simulink library "fzgbib"  (Simulink 4.1.1)
values from neighbouring files (symbols this model uses):
  a_Fzg_max = 2    [PedalInterp_para.m]
  a_Fzg_min = -2    [PedalInterp_para.m]
  gang0 = 1    [PedalInterp_para.m]
  gang_vec = [1 2 3 4]    [PedalInterp_para.m]
  lambda_gang = [1.3 1.25  1.17  1.05]    [PedalInterp_para.m]
  M_Br_max = 4000    [PedalInterp_para.m]
undefined symbols (not defined in the file or in its folder): A, cw, gang, i_d, i_g, m_ab_100pro, m_ab_70pro, m_Fzg, M_mot_max, M_mot_min, n_mot0, n_mot_max, n_mot_min, p_anteil, r_dyn, rho, t_sch, v_bereich, v_Fzg_ms0
libraries: simulink3 x1
(part 1 of 2)
settings Model: LastModifiedBy=MCONRAD

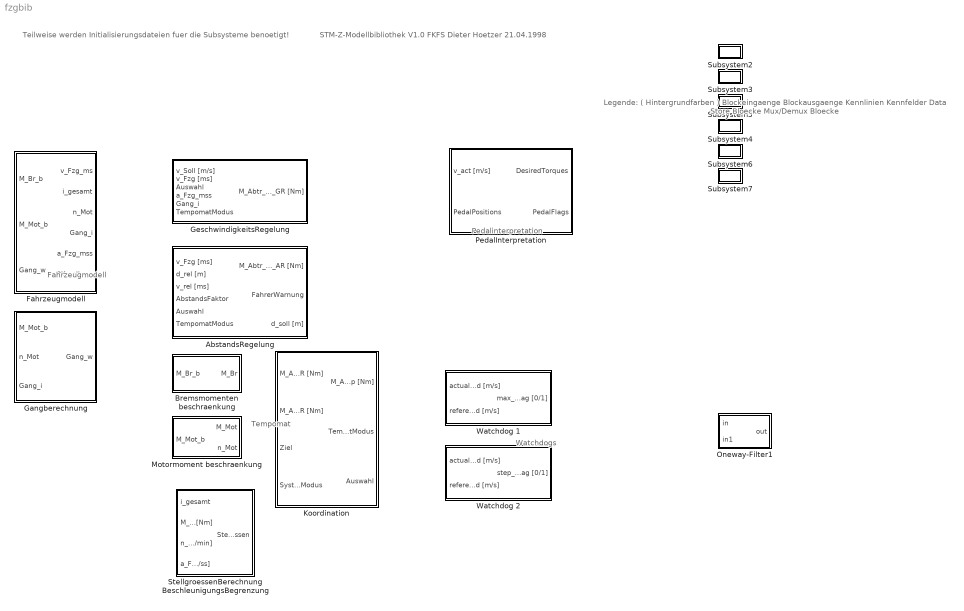
== system fzgbib ==
  note: STM-Z-Modellbibliothek V1.0
      | FKFS
      | Dieter Hoetzer
      | 21.04.1998
  note: Legende:         ( Hintergrundfarben )
      |
      |
      |                      Blockeingaenge
      |
      |                     Blockausgaenge
      |
      |                    Kennlinien
      |
      |                     Kennfelder
      |
      |                     Data Store Bloecke
      |
      |                     Mux/Demux Bloecke
  note: Fahrzeugmodell
  note: Tempomat
  note: Pedalinterpretation
  note: Watchdogs
  note: Teilweise werden Initialisierungsdateien fuer
      | die Subsysteme benoetigt!
  AbstandsRegelung : Subsystem
      settings: RTWFcnNameOpts=Auto  RTWFileNameOpts=Auto
  Bremsmomenten beschraenkung : Subsystem  Orientation=left
      settings: RTWFcnNameOpts=Auto  RTWFileNameOpts=Auto
  Fahrzeugmodell : Subsystem
      settings: RTWFcnNameOpts=Auto  RTWFileNameOpts=Auto
  Gangberechnung : Subsystem
      settings: RTWFcnNameOpts=Auto  RTWFileNameOpts=Auto
  GeschwindigkeitsRegelung : Subsystem
      settings: RTWFcnNameOpts=Auto  RTWFileNameOpts=Auto
  Koordination : Subsystem
      settings: RTWFcnNameOpts=Auto  RTWFileNameOpts=Auto
  Motormoment beschraenkung : Subsystem  Orientation=left
      settings: RTWFcnNameOpts=Auto  RTWFileNameOpts=Auto
  Oneway-Filter1 : Subsystem  mask(Oneway Filter){zk=2}
      mask prompts: zk "Filterkonstante"
      mask help: Filtert Signal mit Zeitkonstante zk nur, wenn kein Sprung auf Null von oben.
      settings: RTWFcnNameOpts=Auto  RTWFileNameOpts=Auto
      mask Display: plot(0,0,100,100,[0 10 20 30 40 50 60 60 100],[0 0 30 50 60 65 67 0 0])
  PedalInterpretation : Subsystem
      settings: RTWFcnNameOpts=Auto  RTWFileNameOpts=Auto
  StellgroessenBerechnung BeschleunigungsBegrenzung : Subsystem
      settings: RTWFcnNameOpts=Auto  RTWFileNameOpts=Auto
  Subsystem2 : Subsystem
      settings: RTWFcnNameOpts=Auto  RTWFileNameOpts=Auto
  Subsystem3 : Subsystem
      settings: RTWFcnNameOpts=Auto  RTWFileNameOpts=Auto
  Subsystem4 : Subsystem
      settings: RTWFcnNameOpts=Auto  RTWFileNameOpts=Auto
  Subsystem5 : Subsystem
      settings: RTWFcnNameOpts=Auto  RTWFileNameOpts=Auto
  Subsystem6 : Subsystem
      settings: RTWFcnNameOpts=Auto  RTWFileNameOpts=Auto
  Subsystem7 : Subsystem
      settings: RTWFcnNameOpts=Auto  RTWFileNameOpts=Auto
  Watchdog 1 : Subsystem
      settings: RTWFcnNameOpts=Auto  RTWFileNameOpts=Auto
  Watchdog 2 : Subsystem
      settings: RTWFcnNameOpts=Auto  RTWFileNameOpts=Auto

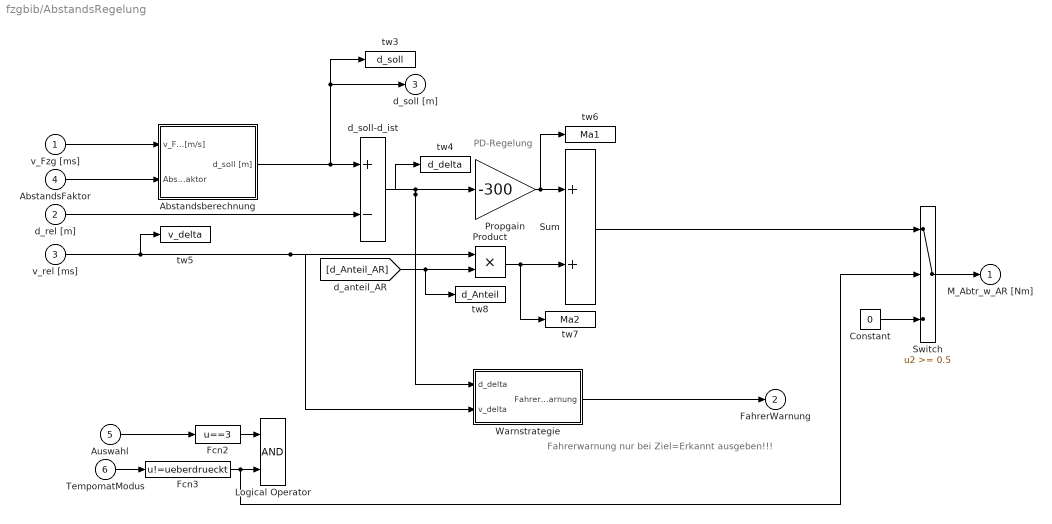
== system fzgbib/AbstandsRegelung ==
  note: PD-Regelung
  note: Fahrerwarnung
      | nur bei Ziel=Erkannt
      | ausgeben!!!
  v_Fzg [ms] : Inport  Port=1  LatchInput=off
  d_rel [m] : Inport  Port=2  LatchInput=off
  v_rel [ms] : Inport  Port=3  LatchInput=off
  AbstandsFaktor : Inport  Port=4  LatchInput=off
  Auswahl : Inport  Port=5  LatchInput=off
  TempomatModus : Inport  Port=6  LatchInput=off
  "Abstandsberechnung " : Subsystem
      settings: RTWFcnNameOpts=Auto  RTWFileNameOpts=Auto
  Constant : Constant  Value=0
  Fcn2 : Fcn  Expr=u==3
  Fcn3 : Fcn  Expr=u!=ueberdrueckt
  Logical Operator : Logic  Operator=AND  Inputs=2
  Product : Product  Inputs=2  Multiplication=Element-wise(.*)  SaturateOnIntegerOverflow=on
  Propgain : Gain  Gain=-300  Multiplication=Element-wise(K.*u)  SaturateOnIntegerOverflow=on
  Sum : Sum  Inputs=++  SaturateOnIntegerOverflow=on
  Switch : Switch  Threshold=0.5
  Warnstrategie : Subsystem
      settings: RTWFcnNameOpts=Auto  RTWFileNameOpts=Auto
  d_soll-d_ist : Sum  Inputs=+-  SaturateOnIntegerOverflow=on
  tw3 : ToWorkspace  VariableName=d_soll  SampleTime=0  SaveFormat=Array
      settings: MaxDataPoints=speicher
  tw4 : ToWorkspace  VariableName=d_delta  SampleTime=0  SaveFormat=Array
      settings: MaxDataPoints=speicher
  tw5 : ToWorkspace  VariableName=v_delta  SampleTime=0  SaveFormat=Array
      settings: MaxDataPoints=speicher
  tw6 : ToWorkspace  VariableName=Ma1  SampleTime=0  SaveFormat=Array
      settings: MaxDataPoints=speicher
  tw7 : ToWorkspace  VariableName=Ma2  SampleTime=0  SaveFormat=Array
      settings: MaxDataPoints=speicher
  tw8 : ToWorkspace  VariableName=d_Anteil  SampleTime=0  SaveFormat=Array
      settings: MaxDataPoints=speicher
  M_Abtr_w_AR [Nm] : Outport  Port=1  InitialOutput=0
  FahrerWarnung : Outport  Port=2  InitialOutput=0
  d_soll [m] : Outport  Port=3  InitialOutput=0
  wires:
  Fcn3/1 -> Switch/2, Logical Operator/2
  TempomatModus/1 -> Fcn3/1
  Fcn2/1 -> Logical Operator/1
  Auswahl/1 -> Fcn2/1
  Sum/1 -> Switch/1
  Switch/1 -> M_Abtr_w_AR [Nm]/1
  Constant/1 -> Switch/3
  Product/1 -> Sum/2, tw7/1
  Propgain/1 -> tw6/1, Sum/1
  d_soll-d_ist/1 -> tw4/1, Propgain/1, Warnstrategie/1(d_delta)
  Warnstrategie/1(FahrerWarnung) -> FahrerWarnung/1
  "Abstandsberechnung "/1(d_soll [m]) -> d_soll-d_ist/1, d_soll [m]/1, tw3/1
  d_rel [m]/1 -> d_soll-d_ist/2
  v_Fzg [ms]/1 -> "Abstandsberechnung "/1(v_Fzg [m/s])
  AbstandsFaktor/1 -> "Abstandsberechnung "/2(AbstandsFaktor)
  v_rel [ms]/1 -> tw5/1, Product/1, Warnstrategie/2(v_delta)
  [d_Anteil_AR] -> Product/2, tw8/1

== system fzgbib/Bremsmomenten beschraenkung ==
  M_Br : Inport  Port=1  LatchInput=off
  Maximales  Bremsmoment : Saturate  UpperLimit=M_Br_max  LowerLimit=0  LinearizeAsGain=on
  M_Br_b : Outport  Port=1  InitialOutput=0
  wires:
  M_Br/1 -> Maximales  Bremsmoment/1
  Maximales  Bremsmoment/1 -> M_Br_b/1

== system fzgbib/Fahrzeugmodell ==
  M_Br_b : Inport  Port=1  LatchInput=off
  M_Mot_b : Inport  Port=2  LatchInput=off
  Gang_w : Inport  Port=3  LatchInput=off
  Drosselklappenstellung : Subsystem
      settings: RTWFcnNameOpts=Auto  RTWFileNameOpts=Auto
  Fahrwiderstaende : Subsystem
      settings: RTWFcnNameOpts=Auto  RTWFileNameOpts=Auto
  Fahrzeugdynamik : Subsystem
      settings: RTWFcnNameOpts=Auto  RTWFileNameOpts=Auto
  tw6 : ToWorkspace  VariableName=v_Fzg_kmh  SampleTime=0  SaveFormat=Array
      settings: MaxDataPoints=speicher
  v_Fzg_ms : Outport  Port=1  InitialOutput=0
  i_gesamt : Outport  Port=2  InitialOutput=0
  n_Mot : Outport  Port=3  InitialOutput=0
  Gang_i : Outport  Port=4  InitialOutput=0
  a_Fzg_mss : Outport  Port=5  InitialOutput=0
  "DK_Stellung " : Outport  Port=6  InitialOutput=0
  wires:
  Fahrwiderstaende/5(i_gesamt) -> i_gesamt/1, Fahrzeugdynamik/5(i_gesamt)
  M_Br_b/1 -> Fahrwiderstaende/2(M_Br_b)
  Gang_w/1 -> Fahrwiderstaende/3(Gang_w)
  M_Mot_b/1 -> Fahrwiderstaende/1(M_Mot_b), Drosselklappenstellung/2(M_Mot_b)
  Fahrwiderstaende/3(F_R) -> Fahrzeugdynamik/3(F_R)
  Fahrwiderstaende/2(F_L) -> Fahrzeugdynamik/2(F_L)
  Fahrwiderstaende/4(F_Brems) -> Fahrzeugdynamik/4(F_Brems)
  Fahrwiderstaende/1(F_A) -> Fahrzeugdynamik/1(F_A)
  Drosselklappenstellung/1(DK_Stellung [Grad]) -> "DK_Stellung "/1
  Fahrzeugdynamik/2(v_Fzg_ms) -> v_Fzg_ms/1, Fahrwiderstaende/4(v_Fzg_ms)
  Fahrzeugdynamik/3(n_Mot) -> n_Mot/1, Drosselklappenstellung/1(n_mot)
  Fahrwiderstaende/6(Gang_i) -> Fahrzeugdynamik/6(Gang_i), Gang_i/1
  Fahrzeugdynamik/1(v_Fzg_kmh) -> tw6/1
  Fahrzeugdynamik/4(a_Fzg_mss) -> a_Fzg_mss/1
  Fahrwiderstaende/7(schalt_l) -> Drosselklappenstellung/3(schalt_l)

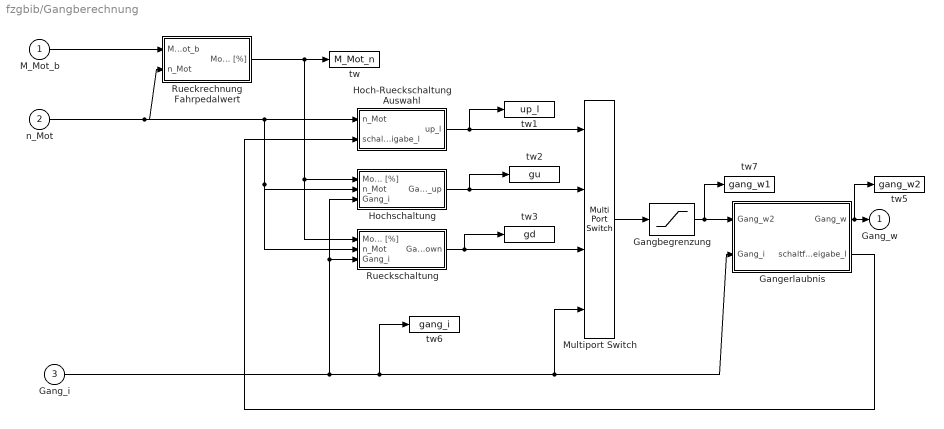
== system fzgbib/Gangberechnung ==
  M_Mot_b : Inport  Port=1  LatchInput=off
  n_Mot : Inport  Port=2  LatchInput=off
  Gang_i : Inport  Port=3  LatchInput=off
  Gangbegrenzung : Saturate  UpperLimit=4  LowerLimit=1  LinearizeAsGain=on
  Gangerlaubnis : Subsystem
      settings: RTWFcnNameOpts=Auto  RTWFileNameOpts=Auto
  Hoch-Rueckschaltung Auswahl : Subsystem
      settings: RTWFcnNameOpts=Auto  RTWFileNameOpts=Auto
  Hochschaltung : Subsystem
      settings: RTWFcnNameOpts=Auto  RTWFileNameOpts=Auto
  Multiport Switch : MultiPortSwitch  Inputs=3
  Rueckrechnung Fahrpedalwert : Subsystem
      settings: RTWFcnNameOpts=Auto  RTWFileNameOpts=Auto
  Rueckschaltung : Subsystem
      settings: RTWFcnNameOpts=Auto  RTWFileNameOpts=Auto
  tw : ToWorkspace  VariableName=M_Mot_n  SampleTime=0  SaveFormat=Array
      settings: MaxDataPoints=speicher
  tw1 : ToWorkspace  VariableName=up_l  SampleTime=0  SaveFormat=Array
      settings: MaxDataPoints=speicher
  tw2 : ToWorkspace  VariableName=gu  SampleTime=0  SaveFormat=Array
      settings: MaxDataPoints=speicher
  tw3 : ToWorkspace  VariableName=gd  SampleTime=0  SaveFormat=Array
      settings: MaxDataPoints=speicher
  tw5 : ToWorkspace  VariableName=gang_w2  SampleTime=0  SaveFormat=Array
      settings: MaxDataPoints=speicher
  tw6 : ToWorkspace  VariableName=gang_i  SampleTime=0  SaveFormat=Array
      settings: MaxDataPoints=speicher
  tw7 : ToWorkspace  VariableName=gang_w1  SampleTime=0  SaveFormat=Array
      settings: MaxDataPoints=speicher
  Gang_w : Outport  Port=1  InitialOutput=0
  wires:
  Gang_i/1 -> tw6/1, Multiport Switch/4, Gangerlaubnis/2(Gang_i), Rueckschaltung/3(Gang_i), Hochschaltung/3(Gang_i)
  Gangerlaubnis/2(schaltfreigabe_l) -> Hoch-Rueckschaltung Auswahl/2(schaltfreigabe_l)
  Gangbegrenzung/1 -> tw7/1, Gangerlaubnis/1(Gang_w2)
  Hoch-Rueckschaltung Auswahl/1(up_l) -> tw1/1, Multiport Switch/1
  Hochschaltung/1(Gang_up) -> tw2/1, Multiport Switch/2
  Gangerlaubnis/1(Gang_w) -> tw5/1, Gang_w/1
  Multiport Switch/1 -> Gangbegrenzung/1
  M_Mot_b/1 -> Rueckrechnung Fahrpedalwert/1(M_Mot_b)
  n_Mot/1 -> Rueckrechnung Fahrpedalwert/2(n_Mot), Hoch-Rueckschaltung Auswahl/1(n_Mot), Hochschaltung/2(n_Mot), Rueckschaltung/2(n_Mot)
  Rueckrechnung Fahrpedalwert/1(Motormoment [%]) -> tw/1, Hochschaltung/1(Motormoment [%]), Rueckschaltung/1(Motormoment [%])
  Rueckschaltung/1(Gang_down) -> Multiport Switch/3, tw3/1

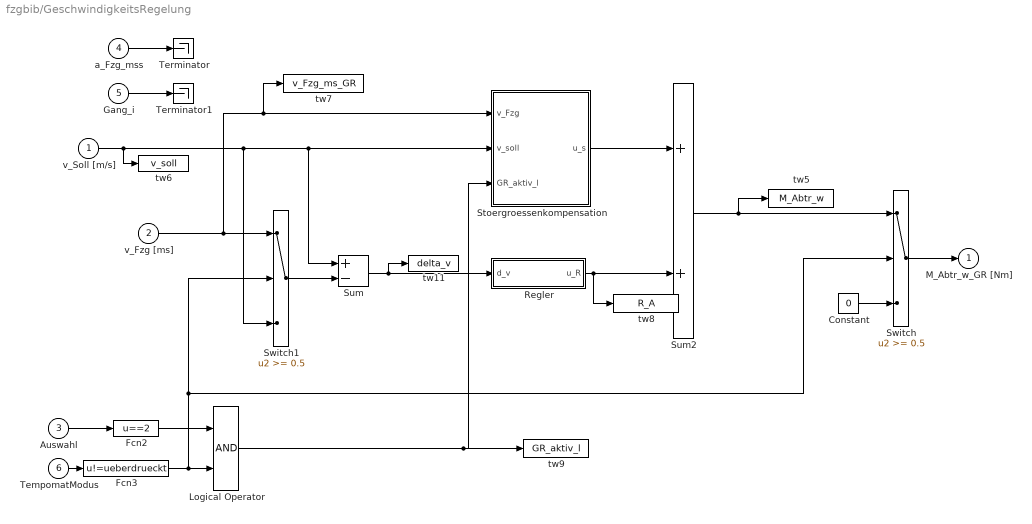
== system fzgbib/GeschwindigkeitsRegelung ==
  v_Soll [m/s] : Inport  Port=1  LatchInput=off
  v_Fzg [ms] : Inport  Port=2  LatchInput=off
  Auswahl : Inport  Port=3  LatchInput=off
  a_Fzg_mss : Inport  Port=4  LatchInput=off
  Gang_i : Inport  Port=5  LatchInput=off
  TempomatModus : Inport  Port=6  LatchInput=off
  Constant : Constant  Value=0
  Fcn2 : Fcn  Expr=u==2
  Fcn3 : Fcn  Expr=u!=ueberdrueckt
  Logical Operator : Logic  Operator=AND  Inputs=2
  Regler : Subsystem
      settings: RTWFcnNameOpts=Auto  RTWFileNameOpts=Auto
  Stoergroessenkompensation : Subsystem
      settings: RTWFcnNameOpts=Auto  RTWFileNameOpts=Auto
  Sum : Sum  Inputs=+-  SaturateOnIntegerOverflow=on
  Sum2 : Sum  Inputs=2  SaturateOnIntegerOverflow=on
  Switch : Switch  Threshold=0.5
  Switch1 : Switch  Threshold=0.5
  Terminator : Terminator
  Terminator1 : Terminator
  tw11 : ToWorkspace  VariableName=delta_v  SampleTime=0  SaveFormat=Array
      settings: MaxDataPoints=speicher
  tw5 : ToWorkspace  VariableName=M_Abtr_w  SampleTime=0  SaveFormat=Array
      settings: MaxDataPoints=speicher
  tw6 : ToWorkspace  VariableName=v_soll  SampleTime=0  SaveFormat=Array
      settings: MaxDataPoints=speicher
  tw7 : ToWorkspace  VariableName=v_Fzg_ms_GR  SampleTime=0  SaveFormat=Array
      settings: MaxDataPoints=speicher
  tw8 : ToWorkspace  VariableName=R_A  SampleTime=0  SaveFormat=Array
      settings: MaxDataPoints=speicher
  tw9 : ToWorkspace  VariableName=GR_aktiv_l  SampleTime=0  SaveFormat=Array
      settings: MaxDataPoints=speicher
  M_Abtr_w_GR [Nm] : Outport  Port=1  InitialOutput=0
  wires:
  v_Soll [m/s]/1 -> Stoergroessenkompensation/2(v_soll), Sum/1, Switch1/3, tw6/1
  Sum2/1 -> tw5/1, Switch/1
  Switch/1 -> M_Abtr_w_GR [Nm]/1
  Fcn3/1 -> Switch/2, Switch1/2, Logical Operator/2
  TempomatModus/1 -> Fcn3/1
  Auswahl/1 -> Fcn2/1
  Fcn2/1 -> Logical Operator/1
  Switch1/1 -> Sum/2
  Constant/1 -> Switch/3
  Sum/1 -> Regler/1(d_v), tw11/1
  v_Fzg [ms]/1 -> Switch1/1, Stoergroessenkompensation/1(v_Fzg), tw7/1
  Stoergroessenkompensation/1(u_s) -> Sum2/1
  a_Fzg_mss/1 -> Terminator/1
  Gang_i/1 -> Terminator1/1
  Regler/1("u_R ") -> Sum2/2, tw8/1
  Logical Operator/1 -> Stoergroessenkompensation/3(GR_aktiv_l), tw9/1

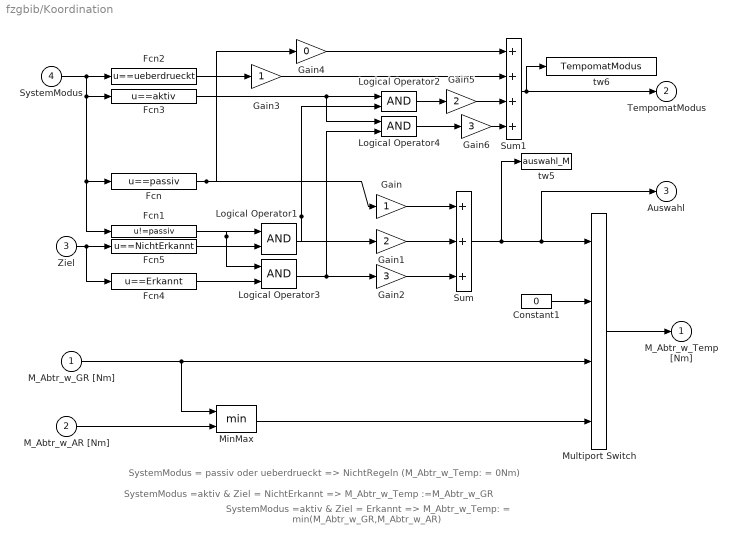
== system fzgbib/Koordination ==
  note: SystemModus = passiv oder ueberdrueckt => NichtRegeln (M_Abtr_w_Temp: = 0Nm)
  note: SystemModus =aktiv & Ziel = Erkannt => M_Abtr_w_Temp: = min(M_Abtr_w_GR,M_Abtr_w_AR)
  note: SystemModus =aktiv & Ziel = NichtErkannt => M_Abtr_w_Temp :=M_Abtr_w_GR
  M_Abtr_w_GR [Nm] : Inport  Port=1  LatchInput=off
  M_Abtr_w_AR [Nm] : Inport  Port=2  LatchInput=off
  Ziel : Inport  Port=3  LatchInput=off
  SystemModus : Inport  Port=4  LatchInput=off
  Constant1 : Constant  Value=0
  Fcn : Fcn  Expr=u==passiv
  Fcn1 : Fcn  Expr=u!=passiv
  Fcn2 : Fcn  Expr=u==ueberdrueckt
  Fcn3 : Fcn  Expr=u==aktiv
  Fcn4 : Fcn  Expr=u==Erkannt
  Fcn5 : Fcn  Expr=u==NichtErkannt
  Gain : Gain  Gain=1  Multiplication=Element-wise(K.*u)  SaturateOnIntegerOverflow=on
  Gain1 : Gain  Gain=2  Multiplication=Element-wise(K.*u)  SaturateOnIntegerOverflow=on
  Gain2 : Gain  Gain=3  Multiplication=Element-wise(K.*u)  SaturateOnIntegerOverflow=on
  Gain3 : Gain  Gain=1  Multiplication=Element-wise(K.*u)  SaturateOnIntegerOverflow=on
  Gain4 : Gain  Gain=0  Multiplication=Element-wise(K.*u)  SaturateOnIntegerOverflow=on
  Gain5 : Gain  Gain=2  Multiplication=Element-wise(K.*u)  SaturateOnIntegerOverflow=on
  Gain6 : Gain  Gain=3  Multiplication=Element-wise(K.*u)  SaturateOnIntegerOverflow=on
  Logical Operator{1..4} (4 alike) : Logic  Operator=AND  Inputs=2
  MinMax : MinMax  Function=min  Inputs=2
  Multiport Switch : MultiPortSwitch  Inputs=3
  Sum : Sum  Inputs=+++  SaturateOnIntegerOverflow=on
  Sum1 : Sum  Inputs=4  SaturateOnIntegerOverflow=on
  tw5 : ToWorkspace  VariableName=auswahl_M  SampleTime=0  SaveFormat=Array
      settings: MaxDataPoints=speicher
  tw6 : ToWorkspace  VariableName=TempomatModus  SampleTime=0  SaveFormat=Array
      settings: MaxDataPoints=speicher
  M_Abtr_w_Temp [Nm] : Outport  Port=1  InitialOutput=0
  TempomatModus : Outport  Port=2  InitialOutput=0
  Auswahl : Outport  Port=3  InitialOutput=0
  wires:
  M_Abtr_w_GR [Nm]/1 -> MinMax/1, Multiport Switch/3
  SystemModus/1 -> Fcn1/1, Fcn/1, Fcn3/1, Fcn2/1
  Ziel/1 -> Fcn4/1, Fcn5/1
  Logical Operator3/1 -> Logical Operator4/2, Gain2/1
  Fcn3/1 -> Logical Operator2/1, Logical Operator4/1
  Sum/1 -> tw5/1, Multiport Switch/1, Auswahl/1
  Multiport Switch/1 -> M_Abtr_w_Temp [Nm]/1
  MinMax/1 -> Multiport Switch/4
  Constant1/1 -> Multiport Switch/2
  Gain4/1 -> Sum1/1
  Fcn/1 -> Gain4/1, Gain/1
  Gain3/1 -> Sum1/2
  Fcn2/1 -> Gain3/1
  M_Abtr_w_AR [Nm]/1 -> MinMax/2
  Fcn4/1 -> Logical Operator3/2
  Fcn1/1 -> Logical Operator1/1, Logical Operator3/1
  Fcn5/1 -> Logical Operator1/2
  Gain/1 -> Sum/1
  Sum1/1 -> TempomatModus/1, tw6/1
  Gain1/1 -> Sum/2
  Logical Operator1/1 -> Gain1/1, Logical Operator2/2
  Gain2/1 -> Sum/3
  Logical Operator2/1 -> Gain5/1
  Gain5/1 -> Sum1/3
  Logical Operator4/1 -> Gain6/1
  Gain6/1 -> Sum1/4

== system fzgbib/Motormoment beschraenkung ==
  M_Mot : Inport  Port=1  LatchInput=off
  n_Mot : Inport  Port=2  LatchInput=off
  Fcn : Fcn  Expr=u>0
  MinMax : MinMax  Function=min  Inputs=2
  Schleppmoment : Lookup  InputValues=n_mot_min  OutputValues=M_mot_min
  Switch : Switch  Threshold=0.5
  maximales Motormoment : Lookup  InputValues=[0 n_mot_max]  OutputValues=[M_mot_max(1) M_mot_max]
  M_Mot_b : Outport  Port=1  InitialOutput=0
  wires:
  MinMax/1 -> Switch/1
  Fcn/1 -> Switch/2
  M_Mot/1 -> Fcn/1, MinMax/1
  Schleppmoment/1 -> Switch/3
  Switch/1 -> M_Mot_b/1
  n_Mot/1 -> maximales Motormoment/1, Schleppmoment/1
  maximales Motormoment/1 -> MinMax/2

== system fzgbib/Oneway-Filter1 ==
  note: 21.5.1997/Hoetzer/FKFS
  in : Inport  Port=1  LatchInput=off
  in1 : Inport  Port=2  LatchInput=off
  1/T : Fcn  Expr=1/u
  Integrator : Integrator  ExternalReset=none  InitialConditionSource=internal  InitialCondition=0  LimitOutput=off  UpperSaturationLimit=inf  LowerSaturationLimit=-inf  ShowSaturationPort=off  ShowStatePort=off  AbsoluteTolerance=auto
  Product : Product  Inputs=2  Multiplication=Element-wise(.*)  SaturateOnIntegerOverflow=on
  Reglerabweichung : Sum  Inputs=-+  SaturateOnIntegerOverflow=on
  "out " : Outport  Port=1  InitialOutput=0
  wires:
  in1/1 -> 1/T/1
  in/1 -> Reglerabweichung/2
  1/T/1 -> Product/2
  Reglerabweichung/1 -> Product/1
  Product/1 -> Integrator/1
  Integrator/1 -> Reglerabweichung/1, "out "/1

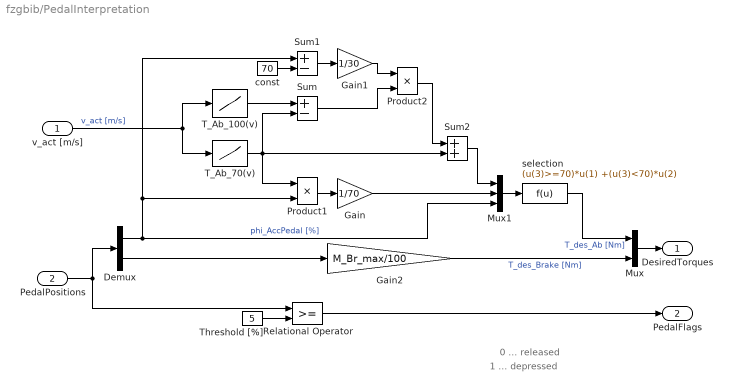
== system fzgbib/PedalInterpretation ==
  note: 1 ... depressed
  note: 0 ... released
  v_act [m/s] : Inport  Port=1  LatchInput=off
  PedalPositions : Inport  Port=2  LatchInput=off
  Demux : Demux  Outputs=2  BusSelectionMode=off
  Gain : Gain  Gain=1/70  Multiplication=Element-wise(K.*u)  SaturateOnIntegerOverflow=on
  Gain1 : Gain  Gain=1/30  Multiplication=Element-wise(K.*u)  SaturateOnIntegerOverflow=on
  Gain2 : Gain  Gain=M_Br_max/100  Multiplication=Element-wise(K.*u)  SaturateOnIntegerOverflow=on
  Mux : Mux  Inputs=2
      settings: DisplayOption=none
  Mux1 : Mux  Inputs=3
      settings: DisplayOption=none
  Product1 : Product  Inputs=2  Multiplication=Element-wise(.*)  SaturateOnIntegerOverflow=on
  Product2 : Product  Inputs=2  Multiplication=Element-wise(.*)  SaturateOnIntegerOverflow=on
  Relational Operator : RelationalOperator  Operator=>=
  Sum : Sum  Inputs=+-  SaturateOnIntegerOverflow=on
  Sum1 : Sum  Inputs=+-  SaturateOnIntegerOverflow=on
  Sum2 : Sum  Inputs=++  SaturateOnIntegerOverflow=on
  T_Ab_100(v) : Lookup  InputValues=v_bereich  OutputValues=m_ab_100pro
  T_Ab_70(v) : Lookup  InputValues=v_bereich  OutputValues=m_ab_70pro
  Threshold [%] : Constant  Value=5
  const : Constant  Value=70
  selection : Fcn  Expr=(u(3)>=70)*u(1) +(u(3)<70)*u(2)
  DesiredTorques : Outport  Port=1  InitialOutput=0
  PedalFlags : Outport  Port=2  InitialOutput=0
  wires:
  Threshold [%]/1 -> Relational Operator/2
  Sum2/1 -> Mux1/1
  Gain/1 -> Mux1/2
  Gain1/1 -> Product2/1
  Sum/1 -> Product2/2
  Sum1/1 -> Gain1/1
  const/1 -> Sum1/2
  selection/1 -> Mux/1  "T_des_Ab [Nm]"
  Mux1/1 -> selection/1
  Demux/1 -> Mux1/3, Sum1/1, Product1/2  "phi_AccPedal [%]"
  PedalPositions/1 -> Relational Operator/1, Demux/1
  Demux/2 -> Gain2/1
  Gain2/1 -> Mux/2  "T_des_Brake [Nm]"
  v_act [m/s]/1 -> T_Ab_100(v)/1, T_Ab_70(v)/1  "v_act [m/s]"
  Product2/1 -> Sum2/1
  T_Ab_70(v)/1 -> Sum2/2, Product1/1, Sum/2
  T_Ab_100(v)/1 -> Sum/1
  Product1/1 -> Gain/1
  Mux/1 -> DesiredTorques/1
  Relational Operator/1 -> PedalFlags/1

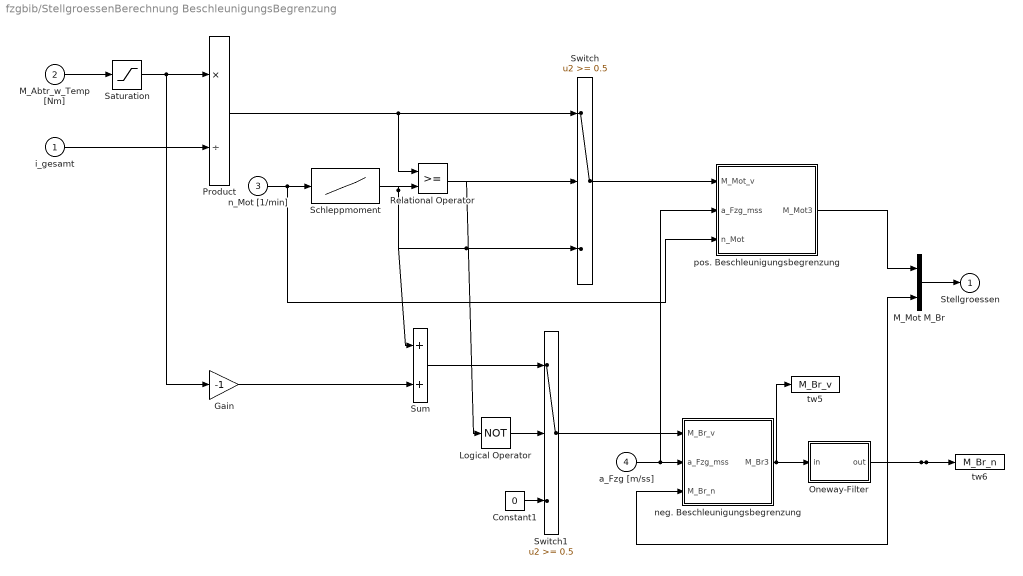
== system fzgbib/StellgroessenBerechnung BeschleunigungsBegrenzung ==
  i_gesamt : Inport  Port=1  LatchInput=off
  M_Abtr_w_Temp [Nm] : Inport  Port=2  LatchInput=off
  "n_Mot [1/min] " : Inport  Port=3  LatchInput=off
  a_Fzg [m/ss] : Inport  Port=4  LatchInput=off
  Constant1 : Constant  Value=0
  Gain : Gain  Gain=-1  Multiplication=Element-wise(K.*u)  SaturateOnIntegerOverflow=on
  Logical Operator : Logic  Operator=NOT  Inputs=1
  M_Mot M_Br : Mux  Inputs=2
      settings: DisplayOption=none
  Oneway-Filter : Subsystem  mask(Oneway Filter){zk=2}
      mask prompts: zk "Filterkonstante"
      mask help: Filtert Signal mit Zeitkonstante zk nur, wenn kein Sprung auf Null von oben.
      settings: RTWFcnNameOpts=Auto  RTWFileNameOpts=Auto
      mask Display: plot(0,0,100,100,[0 10 20 30 40 50 60 60 100],[0 0 30 50 60 65 67 0 0])
  Product : Product  Inputs=*/  Multiplication=Element-wise(.*)  SaturateOnIntegerOverflow=on
  Relational Operator : RelationalOperator  Operator=>=
  Saturation : Saturate  UpperLimit=m_Fzg*a_Fzg_max*r_dyn  LowerLimit=m_Fzg*a_Fzg_min*r_dyn  LinearizeAsGain=on
  Schleppmoment : Lookup  InputValues=n_mot_min  OutputValues=M_mot_min
  Sum : Sum  Inputs=++  SaturateOnIntegerOverflow=on
  Switch : Switch  Threshold=0.5
  Switch1 : Switch  Threshold=0.5
  neg. Beschleunigungsbegrenzung : Subsystem
      settings: RTWFcnNameOpts=Auto  RTWFileNameOpts=Auto
  pos. Beschleunigungsbegrenzung : Subsystem
      settings: RTWFcnNameOpts=Auto  RTWFileNameOpts=Auto
  tw5 : ToWorkspace  VariableName=M_Br_v  SampleTime=0  SaveFormat=Array
      settings: MaxDataPoints=speicher
  tw6 : ToWorkspace  VariableName=M_Br_n  SampleTime=0  SaveFormat=Array
      settings: MaxDataPoints=speicher
  Stellgroessen : Outport  Port=1  InitialOutput=0
  wires:
  Saturation/1 -> Gain/1, Product/1
  M_Abtr_w_Temp [Nm]/1 -> Saturation/1
  Switch1/1 -> neg. Beschleunigungsbegrenzung/1(M_Br_v)
  Product/1 -> Switch/1, Relational Operator/1
  "n_Mot [1/min] "/1 -> pos. Beschleunigungsbegrenzung/3("n_Mot "), Schleppmoment/1
  a_Fzg [m/ss]/1 -> pos. Beschleunigungsbegrenzung/2(a_Fzg_mss), neg. Beschleunigungsbegrenzung/2(a_Fzg_mss)
  pos. Beschleunigungsbegrenzung/1(M_Mot3) -> M_Mot M_Br/1
  Switch/1 -> pos. Beschleunigungsbegrenzung/1(M_Mot_v)
  Sum/1 -> Switch1/1
  Gain/1 -> Sum/2
  i_gesamt/1 -> Product/2
  Oneway-Filter/1("out ") -> neg. Beschleunigungsbegrenzung/3(M_Br_n), tw6/1, M_Mot M_Br/2
  neg. Beschleunigungsbegrenzung/1(M_Br3) -> tw5/1, Oneway-Filter/1(in)
  M_Mot M_Br/1 -> Stellgroessen/1
  Logical Operator/1 -> Switch1/2
  Constant1/1 -> Switch1/3
  Relational Operator/1 -> Switch/2, Logical Operator/1
  Schleppmoment/1 -> Switch/3, Sum/1, Relational Operator/2

== system fzgbib/Subsystem2 ==

== system fzgbib/Subsystem3 ==

== system fzgbib/Subsystem4 ==

== system fzgbib/Subsystem5 ==

== system fzgbib/Subsystem6 ==

== system fzgbib/Subsystem7 ==

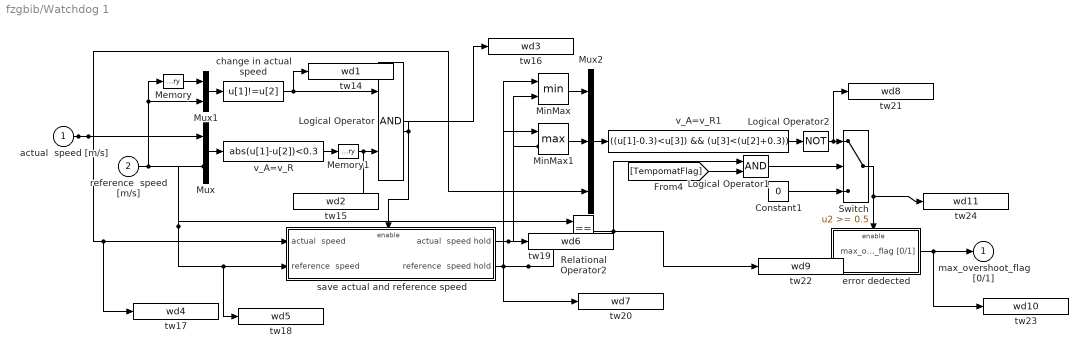
== system fzgbib/Watchdog 1 ==
  actual  speed [m/s] : Inport  Port=1  LatchInput=off
  reference  speed [m/s] : Inport  Port=2  LatchInput=off
  Constant1 : Constant  Value=0
  Logical Operator : Logic  Operator=AND  Inputs=2
  Logical Operator1 : Logic  Operator=AND  Inputs=2
  Logical Operator2 : Logic  Operator=NOT  Inputs=1
  Memory : Memory  X0=0  InheritSampleTime=off
      settings: RTWStateStorageClass=Auto
  Memory1 : Memory  X0=0  InheritSampleTime=off
      settings: RTWStateStorageClass=Auto
  MinMax : MinMax  Function=min  Inputs=2
  MinMax1 : MinMax  Function=max  Inputs=2
  Mux : Mux  Inputs=2
      settings: DisplayOption=none
  Mux1 : Mux  Inputs=2
      settings: DisplayOption=none
  Mux2 : Mux  Inputs=3
      settings: DisplayOption=none
  Relational Operator2 : RelationalOperator  Operator===
  Switch : Switch  Threshold=0.5
  change in actual speed : Fcn  Expr=u[1]!=u[2]
  error dedected : Subsystem  TreatAsAtomicUnit=on
      settings: RTWFcnNameOpts=Auto  RTWFileNameOpts=Auto
  save actual and reference speed : Subsystem  TreatAsAtomicUnit=on
      settings: RTWFcnNameOpts=Auto  RTWFileNameOpts=Auto
  tw14 : ToWorkspace  VariableName=wd1  SampleTime=0  SaveFormat=Array
      settings: MaxDataPoints=speicher
  tw15 : ToWorkspace  VariableName=wd2  SampleTime=0  SaveFormat=Array
      settings: MaxDataPoints=speicher
  tw16 : ToWorkspace  VariableName=wd3  SampleTime=0  SaveFormat=Array
      settings: MaxDataPoints=speicher
  tw17 : ToWorkspace  VariableName=wd4  SampleTime=0  SaveFormat=Array
      settings: MaxDataPoints=speicher
  tw18 : ToWorkspace  VariableName=wd5  SampleTime=0  SaveFormat=Array
      settings: MaxDataPoints=speicher
  tw19 : ToWorkspace  VariableName=wd6  SampleTime=0  SaveFormat=Array
      settings: MaxDataPoints=speicher
  tw20 : ToWorkspace  VariableName=wd7  SampleTime=0  SaveFormat=Array
      settings: MaxDataPoints=speicher
  tw21 : ToWorkspace  VariableName=wd8  SampleTime=0  SaveFormat=Array
      settings: MaxDataPoints=speicher
  tw22 : ToWorkspace  VariableName=wd9  SampleTime=0  SaveFormat=Array
      settings: MaxDataPoints=speicher
  tw23 : ToWorkspace  VariableName=wd10  SampleTime=0  SaveFormat=Array
      settings: MaxDataPoints=speicher
  tw24 : ToWorkspace  VariableName=wd11  SampleTime=0  SaveFormat=Array
      settings: MaxDataPoints=speicher
  v_A=v_R : Fcn  Expr=abs(u[1]-u[2])<0.3
  v_A=v_R1 : Fcn  Expr=((u[1]-0.3)<u[3]) && (u[3]<(u[2]+0.3))
  max_overshoot_flag [0/1] : Outport  Port=1  InitialOutput=0
  wires:
  actual  speed [m/s]/1 -> Mux2/3, Mux/1, save actual and reference speed/1("actual  speed "), tw17/1
  reference  speed [m/s]/1 -> Mux/2, Relational Operator2/1, save actual and reference speed/2("reference  speed  "), tw18/1, Memory/1, Mux1/2
  v_A=v_R/1 -> Memory1/1
  Mux/1 -> v_A=v_R/1
  Memory/1 -> Mux1/1
  Mux1/1 -> change in actual speed/1
  v_A=v_R1/1 -> Logical Operator2/1
  MinMax1/1 -> Mux2/2
  MinMax/1 -> Mux2/1
  Mux2/1 -> v_A=v_R1/1
  Constant1/1 -> Switch/3
  save actual and reference speed/2(reference  speed hold) -> Relational Operator2/2, MinMax/1, MinMax1/1, tw20/1
  change in actual speed/1 -> Logical Operator/1, tw14/1
  Memory1/1 -> Logical Operator/2, tw15/1
  Logical Operator/1 -> save actual and reference speed/Enable, tw16/1
  save actual and reference speed/1(actual  speed hold) -> MinMax/2, MinMax1/2, tw19/1
  Logical Operator2/1 -> Switch/1, tw21/1
  error dedected/1(max_overshoot_flag [0/1]) -> max_overshoot_flag [0/1]/1, tw23/1
  Switch/1 -> error dedected/Enable, tw24/1
  Logical Operator1/1 -> Switch/2
  Relational Operator2/1 -> tw22/1, Logical Operator1/1
  [TempomatFlag] -> Logical Operator1/2

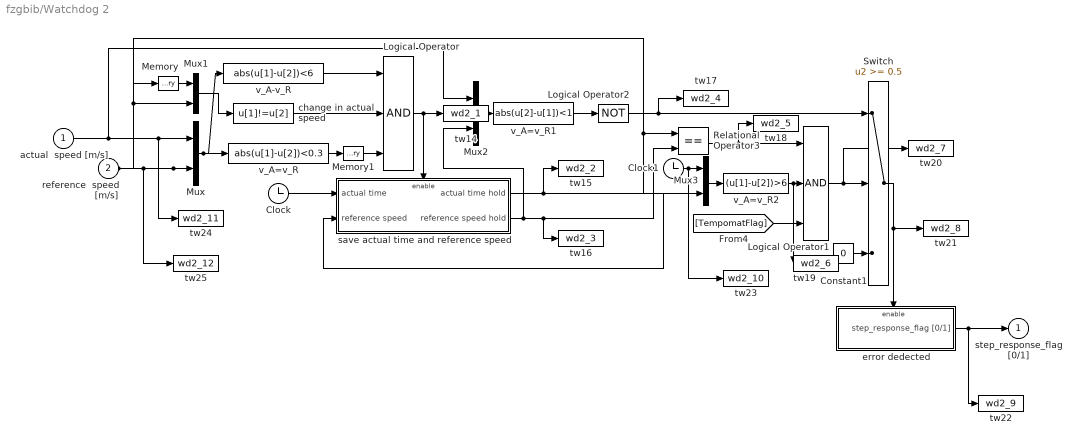
== system fzgbib/Watchdog 2 ==
  actual  speed [m/s] : Inport  Port=1  LatchInput=off
  reference  speed [m/s] : Inport  Port=2  LatchInput=off
  Clock : Clock
      settings: DisplayTime=off  Decimation=10
  Clock1 : Clock
      settings: DisplayTime=off  Decimation=10
  Constant1 : Constant  Value=0
  Logical Operator : Logic  Operator=AND  Inputs=3
  Logical Operator1 : Logic  Operator=AND  Inputs=3
  Logical Operator2 : Logic  Operator=NOT  Inputs=1
  Memory : Memory  X0=0  InheritSampleTime=off
      settings: RTWStateStorageClass=Auto
  Memory1 : Memory  X0=0  InheritSampleTime=off
      settings: RTWStateStorageClass=Auto
  Mux{,1..3} (4 alike) : Mux  Inputs=2
      settings: DisplayOption=none
  Relational Operator3 : RelationalOperator  Operator===
  Switch : Switch  Threshold=0.5
  change in actual speed : Fcn  Expr=u[1]!=u[2]
  error dedected : Subsystem  TreatAsAtomicUnit=on
      settings: RTWFcnNameOpts=Auto  RTWFileNameOpts=Auto
  save actual time and reference speed : Subsystem  TreatAsAtomicUnit=on
      settings: RTWFcnNameOpts=Auto  RTWFileNameOpts=Auto
  tw14 : ToWorkspace  VariableName=wd2_1  SampleTime=0  SaveFormat=Array
      settings: MaxDataPoints=speicher
  tw15 : ToWorkspace  VariableName=wd2_2  SampleTime=0  SaveFormat=Array
      settings: MaxDataPoints=speicher
  tw16 : ToWorkspace  VariableName=wd2_3  SampleTime=0  SaveFormat=Array
      settings: MaxDataPoints=speicher
  tw17 : ToWorkspace  VariableName=wd2_4  SampleTime=0  SaveFormat=Array
      settings: MaxDataPoints=speicher
  tw18 : ToWorkspace  VariableName=wd2_5  SampleTime=0  SaveFormat=Array
      settings: MaxDataPoints=speicher
  tw19 : ToWorkspace  VariableName=wd2_6  SampleTime=0  SaveFormat=Array
      settings: MaxDataPoints=speicher
  tw20 : ToWorkspace  VariableName=wd2_7  SampleTime=0  SaveFormat=Array
      settings: MaxDataPoints=speicher
  tw21 : ToWorkspace  VariableName=wd2_8  SampleTime=0  SaveFormat=Array
      settings: MaxDataPoints=speicher
  tw22 : ToWorkspace  VariableName=wd2_9  SampleTime=0  SaveFormat=Array
      settings: MaxDataPoints=speicher
  tw23 : ToWorkspace  VariableName=wd2_10  SampleTime=0  SaveFormat=Array
      settings: MaxDataPoints=speicher
  tw24 : ToWorkspace  VariableName=wd2_11  SampleTime=0  SaveFormat=Array
      settings: MaxDataPoints=speicher
  tw25 : ToWorkspace  VariableName=wd2_12  SampleTime=0  SaveFormat=Array
      settings: MaxDataPoints=speicher
  v_A-v_R : Fcn  Expr=abs(u[1]-u[2])<6
  v_A=v_R : Fcn  Expr=abs(u[1]-u[2])<0.3
  v_A=v_R1 : Fcn  Expr=abs(u[2]-u[1])<1
  v_A=v_R2 : Fcn  Expr=(u[1]-u[2])>6
  step_response_flag [0/1] : Outport  Port=1  InitialOutput=0
  wires:
  Memory1/1 -> Logical Operator/3
  v_A=v_R/1 -> Memory1/1
  v_A-v_R/1 -> Logical Operator/1
  change in actual speed/1 -> Logical Operator/2
  reference  speed [m/s]/1 -> Mux1/2, Memory/1, Mux/2, save actual time and reference speed/2("reference speed  "), Relational Operator3/1, tw25/1
  Mux/1 -> v_A-v_R/1, v_A=v_R/1
  Mux1/1 -> change in actual speed/1
  Memory/1 -> Mux1/1
  Clock/1 -> save actual time and reference speed/1("actual time ")
  v_A=v_R1/1 -> Logical Operator2/1
  actual  speed [m/s]/1 -> Mux2/1, Mux/1, tw24/1
  Mux2/1 -> v_A=v_R1/1
  save actual time and reference speed/2(reference speed hold) -> Mux2/2, Relational Operator3/2, tw16/1
  Mux3/1 -> v_A=v_R2/1
  Constant1/1 -> Switch/3
  [TempomatFlag] -> Logical Operator1/3
  Logical Operator/1 -> save actual time and reference speed/Enable, tw14/1
  save actual time and reference speed/1(actual time hold) -> Mux3/2, tw15/1
  Logical Operator2/1 -> Switch/1, tw17/1
  Relational Operator3/1 -> Logical Operator1/1, tw18/1
  v_A=v_R2/1 -> Logical Operator1/2, tw19/1
  Logical Operator1/1 -> Switch/2, tw20/1
  Switch/1 -> error dedected/Enable, tw21/1
  error dedected/1(step_response_flag [0/1]) -> step_response_flag [0/1]/1, tw22/1
  Clock1/1 -> Mux3/1, tw23/1

== system fzgbib/AbstandsRegelung/Abstandsberechnung  ==
  note: SollAbstand:= "Tacho halbe" x AbstandsFaktor
  v_Fzg [m/s] : Inport  Port=1  LatchInput=off
  AbstandsFaktor : Inport  Port=2  LatchInput=off
  Gain : Gain  Gain=1.8  Multiplication=Element-wise(K.*u)  SaturateOnIntegerOverflow=on
  Product : Product  Inputs=2  Multiplication=Element-wise(.*)  SaturateOnIntegerOverflow=on
  d_soll [m] : Outport  Port=1
  wires:
  v_Fzg [m/s]/1 -> Gain/1
  AbstandsFaktor/1 -> Product/2
  Gain/1 -> Product/1
  Product/1 -> d_soll [m]/1

== system fzgbib/AbstandsRegelung/Warnstrategie ==
  note: wenn d_ist<d_soll und sich vorderes Fzg weiter naehert
  note: FahrerWarnung :=
      |  (IstAbstand < SollAbstand) & IstAbstand verringert sich
  d_delta : Inport  Port=1  LatchInput=off
  v_delta : Inport  Port=2  LatchInput=off
  Constant : Constant  Value=0
  Logical Operator : Logic  Operator=AND  Inputs=2
  Relational Operator : RelationalOperator  Operator=>
  Relational Operator1 : RelationalOperator  Operator=<
  FahrerWarnung : Outport  Port=1
  wires:
  Constant/1 -> Relational Operator1/2, Relational Operator/2
  d_delta/1 -> Relational Operator/1
  Relational Operator/1 -> Logical Operator/1
  Logical Operator/1 -> FahrerWarnung/1
  v_delta/1 -> Relational Operator1/1
  Relational Operator1/1 -> Logical Operator/2

== system fzgbib/Fahrzeugmodell/Drosselklappenstellung ==
  n_mot : Inport  Port=1  LatchInput=off
  M_Mot_b : Inport  Port=2  LatchInput=off
  schalt_l : Inport  Port=3  LatchInput=off
  Constant : Constant  Value=0
  Constant1 : Constant  Value=n_mot0+100
  Constant2 : Constant  Value=0
  Drosselklappen- kennfeld : simulink3/Functions & Tables/Look-Up Table (2-D)  x=n_Mot_vec  y=M_Mot_vec  t=Drossel_mat
  Logical Operator : Logic  Operator=AND  Inputs=2
  Logical Operator1 : Logic  Operator=OR  Inputs=2
  PT1 Filterung : TransferFcn  Numerator=[1]  Denominator=[0.1 1]  AbsoluteTolerance=auto  Realization=auto
  Relational Operator : RelationalOperator  Operator=>=
  Relational Operator1 : RelationalOperator  Operator=<=
  Saturation : Saturate  UpperLimit=90  LowerLimit=0  LinearizeAsGain=on
  Switch : Switch  Threshold=0.5
  damit bei Vollast 90 Grad : Fcn  Expr=u+3
  DK_Stellung [Grad] : Outport  Port=1  InitialOutput=0
  wires:
  damit bei Vollast 90 Grad/1 -> Switch/3
  Drosselklappen- kennfeld/1 -> damit bei Vollast 90 Grad/1
  n_mot/1 -> Drosselklappen- kennfeld/1, Relational Operator/1
  M_Mot_b/1 -> Drosselklappen- kennfeld/2, Relational Operator1/1
  Switch/1 -> Saturation/1
  PT1 Filterung/1 -> DK_Stellung [Grad]/1
  Saturation/1 -> PT1 Filterung/1
  Constant1/1 -> Relational Operator/2
  Constant2/1 -> Relational Operator1/2
  Logical Operator1/1 -> Switch/2
  Constant/1 -> Switch/1
  schalt_l/1 -> Logical Operator1/2
  Logical Operator/1 -> Logical Operator1/1
  Relational Operator/1 -> Logical Operator/1
  Relational Operator1/1 -> Logical Operator/2

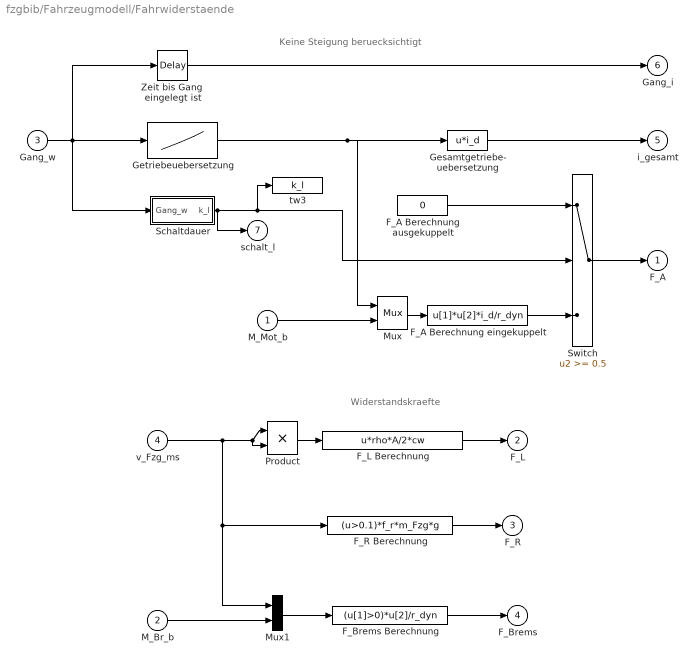
== system fzgbib/Fahrzeugmodell/Fahrwiderstaende ==
  note: Keine Steigung beruecksichtigt
  note: Widerstandskraefte
  M_Mot_b : Inport  Port=1  LatchInput=off
  M_Br_b : Inport  Port=2  LatchInput=off
  Gang_w : Inport  Port=3  LatchInput=off
  v_Fzg_ms : Inport  Port=4  LatchInput=off
  F_A Berechnung ausgekuppelt : Constant  Value=0
  F_A Berechnung eingekuppelt : Fcn  Expr=u[1]*u[2]*i_d/r_dyn
  F_Brems Berechnung : Fcn  Expr=(u[1]>0)*u[2]/r_dyn
  F_L Berechnung : Fcn  Expr=u*rho*A/2*cw
  F_R Berechnung : Fcn  Expr=(u>0.1)*f_r*m_Fzg*g
  Gesamtgetriebe- uebersetzung : Fcn  Expr=u*i_d
  Getriebeuebersetzung : Lookup  InputValues=gang  OutputValues=i_g
  Mux : Mux  Inputs=2
      settings: DisplayOption=none
  Mux1 : Mux  Inputs=2
      settings: DisplayOption=none
  Product : Product  Inputs=2  Multiplication=Element-wise(.*)  SaturateOnIntegerOverflow=on
  Schaltdauer : Subsystem
      settings: RTWFcnNameOpts=Auto  RTWFileNameOpts=Auto
  Switch : Switch  Threshold=0.5
  Zeit bis Gang  eingelegt ist : TransportDelay  DelayTime=t_sch  InitialInput=1  BufferSize=1024  PadeOrder=0
  tw3 : ToWorkspace  VariableName=k_l  SampleTime=0  SaveFormat=Array
      settings: MaxDataPoints=speicher
  F_A : Outport  Port=1  InitialOutput=0
  F_L : Outport  Port=2  InitialOutput=0
  F_R : Outport  Port=3  InitialOutput=0
  F_Brems : Outport  Port=4  InitialOutput=0
  i_gesamt : Outport  Port=5  InitialOutput=0
  Gang_i : Outport  Port=6  InitialOutput=0
  schalt_l : Outport  Port=7  InitialOutput=0
  wires:
  Zeit bis Gang  eingelegt ist/1 -> Gang_i/1
  F_A Berechnung ausgekuppelt/1 -> Switch/1
  Gang_w/1 -> Zeit bis Gang  eingelegt ist/1, Schaltdauer/1(Gang_w), Getriebeuebersetzung/1
  Switch/1 -> F_A/1
  Getriebeuebersetzung/1 -> Gesamtgetriebe- uebersetzung/1, Mux/1
  Gesamtgetriebe- uebersetzung/1 -> i_gesamt/1
  Mux/1 -> F_A Berechnung eingekuppelt/1
  M_Mot_b/1 -> Mux/2
  F_A Berechnung eingekuppelt/1 -> Switch/3
  Schaltdauer/1(k_l) -> tw3/1, Switch/2, schalt_l/1
  M_Br_b/1 -> Mux1/2
  Mux1/1 -> F_Brems Berechnung/1
  F_R Berechnung/1 -> F_R/1
  F_Brems Berechnung/1 -> F_Brems/1
  v_Fzg_ms/1 -> Mux1/1, F_R Berechnung/1, Product/1, Product/2
  Product/1 -> F_L Berechnung/1
  F_L Berechnung/1 -> F_L/1

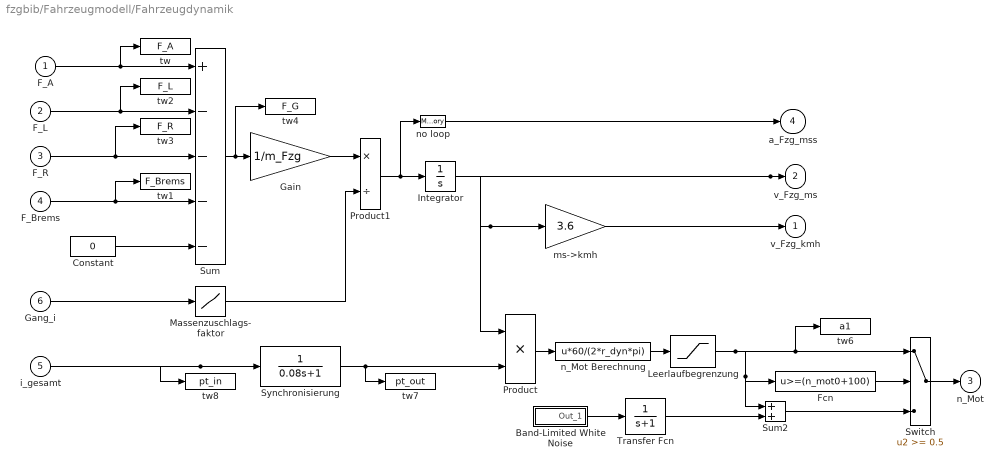
== system fzgbib/Fahrzeugmodell/Fahrzeugdynamik ==
  F_A : Inport  Port=1  LatchInput=off
  F_L : Inport  Port=2  LatchInput=off
  F_R : Inport  Port=3  LatchInput=off
  F_Brems : Inport  Port=4  LatchInput=off
  i_gesamt : Inport  Port=5  LatchInput=off
  Gang_i : Inport  Port=6  LatchInput=off
  Band-Limited White Noise : Subsystem  mask(Continuous White Noise.){@1=[3], @2=0.2, @3=[23341]}
      mask prompts: @1 "Noise Power:"; @2 "Sample Time:"; @3 "Seed"
      mask help:
      | White noise for continuous (s-domain) systems.
      | Band-limited using zero-order-hold.
      mask init:
      | Cov = @1; Ts = @2; seed = @3; r = rand(1,12); r2 = [r(1),r;r,r(12)]; t =[1:13;1:13];
      settings: RTWFcnNameOpts=Auto  RTWFileNameOpts=Auto
      mask Help: Implemented using white noise into Zero-Order Hold block. The seed and power can be vectors of the same length to produce a vector of white noise sources. For faster simulation, set sample time to the highest value possible but in accordance with the fastest dynamics of system.
      mask Display: plot(t(:),r2(:))
  Constant : Constant  Value=0
  Fcn : Fcn  Expr=u>=(n_mot0+100)
  Gain : Gain  Gain=1/m_Fzg  Multiplication=Element-wise(K.*u)  SaturateOnIntegerOverflow=on
  Integrator : Integrator  ExternalReset=none  InitialConditionSource=internal  InitialCondition=v_Fzg_ms0  LimitOutput=off  UpperSaturationLimit=100  LowerSaturationLimit=0  ShowSaturationPort=off  ShowStatePort=off  AbsoluteTolerance=auto
  Leerlaufbegrenzung : Saturate  UpperLimit=7000  LowerLimit=n_mot0  LinearizeAsGain=on
  Massenzuschlags- faktor : Lookup  InputValues=gang_vec  OutputValues=lambda_gang
  Product : Product  Inputs=2  Multiplication=Element-wise(.*)  SaturateOnIntegerOverflow=on
  Product1 : Product  Inputs=*/  Multiplication=Element-wise(.*)  SaturateOnIntegerOverflow=on
  Sum : Sum  Inputs=+----  SaturateOnIntegerOverflow=on
  Sum2 : Sum  Inputs=++  SaturateOnIntegerOverflow=on
  Switch : Switch  Threshold=0.5
  Synchronisierung : TransferFcn  Numerator=[1]  Denominator=[0.08 1]  AbsoluteTolerance=auto  Realization=auto
  Transfer Fcn : TransferFcn  Numerator=[1]  Denominator=[1 1]  AbsoluteTolerance=auto  Realization=auto
  ms->kmh : Gain  Gain=3.6  Multiplication=Element-wise(K.*u)  SaturateOnIntegerOverflow=on
  n_Mot Berechnung : Fcn  Expr=u*60/(2*r_dyn*pi)
  no loop : Memory  X0=0  InheritSampleTime=off
      settings: RTWStateStorageClass=Auto
  tw : ToWorkspace  VariableName=F_A  SampleTime=0  SaveFormat=Array
      settings: MaxDataPoints=speicher
  tw1 : ToWorkspace  VariableName=F_Brems  SampleTime=0  SaveFormat=Array
      settings: MaxDataPoints=speicher
  tw2 : ToWorkspace  VariableName=F_L  SampleTime=0  SaveFormat=Array
      settings: MaxDataPoints=speicher
  tw3 : ToWorkspace  VariableName=F_R  SampleTime=0  SaveFormat=Array
      settings: MaxDataPoints=speicher
  tw4 : ToWorkspace  VariableName=F_G  SampleTime=0  SaveFormat=Array
      settings: MaxDataPoints=speicher
  tw6 : ToWorkspace  VariableName=a1  SampleTime=0  SaveFormat=Array
      settings: MaxDataPoints=speicher
  tw7 : ToWorkspace  VariableName=pt_out  SampleTime=0  SaveFormat=Array
      settings: MaxDataPoints=speicher
  tw8 : ToWorkspace  VariableName=pt_in  SampleTime=0  SaveFormat=Array
      settings: MaxDataPoints=speicher
  v_Fzg_kmh : Outport  Port=1  InitialOutput=0
  v_Fzg_ms : Outport  Port=2  InitialOutput=0
  n_Mot : Outport  Port=3  InitialOutput=0
  a_Fzg_mss : Outport  Port=4  InitialOutput=0
  wires:
  Switch/1 -> n_Mot/1
  Band-Limited White Noise/1(Out_1) -> Transfer Fcn/1
  Transfer Fcn/1 -> Sum2/2
  Leerlaufbegrenzung/1 -> Fcn/1, Sum2/1, Switch/1, tw6/1
  Sum2/1 -> Switch/3
  Fcn/1 -> Switch/2
  i_gesamt/1 -> tw8/1, Synchronisierung/1
  Synchronisierung/1 -> tw7/1, Product/2
  Sum/1 -> tw4/1, Gain/1
  Gain/1 -> Product1/1
  Product1/1 -> Integrator/1, no loop/1
  Massenzuschlags- faktor/1 -> Product1/2
  Gang_i/1 -> Massenzuschlags- faktor/1
  n_Mot Berechnung/1 -> Leerlaufbegrenzung/1
  Product/1 -> n_Mot Berechnung/1
  no loop/1 -> a_Fzg_mss/1
  Integrator/1 -> v_Fzg_ms/1, ms->kmh/1, Product/1
  ms->kmh/1 -> v_Fzg_kmh/1
  F_A/1 -> Sum/1, tw/1
  F_L/1 -> tw2/1, Sum/2
  F_R/1 -> tw3/1, Sum/3
  F_Brems/1 -> Sum/4, tw1/1
  Constant/1 -> Sum/5

== system fzgbib/Gangberechnung/Gangerlaubnis ==
  Gang_w2 : Inport  Port=1  LatchInput=off
  Gang_i : Inport  Port=2  LatchInput=off
  == : RelationalOperator  Operator===
  Gangspeicher : Memory  X0=gang0  InheritSampleTime=off
      settings: RTWStateStorageClass=Auto
  Switch : Switch  Threshold=0.5
  Gang_w : Outport  Port=1  InitialOutput=0
  schaltfreigabe_l : Outport  Port=2  InitialOutput=0
  wires:
  Gang_i/1 -> ==/1
  Gang_w2/1 -> Switch/1
  ==/1 -> schaltfreigabe_l/1, Switch/2
  Switch/1 -> Gangspeicher/1
  Gangspeicher/1 -> Gang_w/1, Switch/3, ==/2

== system fzgbib/Gangberechnung/Hoch-Rueckschaltung Auswahl ==
  n_Mot : Inport  Port=1  LatchInput=off
  schaltfreigabe_l : Inport  Port=2  LatchInput=off
  Clock1 : Clock
      settings: DisplayTime=off  Decimation=10
  Data Store : DataStoreMemory  DataStoreName=time1  InitialValue=0
  Fcn : Fcn  Expr=(u[2]==1)*((u[1]>=0)*1+(u[1]<0)*2)+(u[2]==0)*3
  Fcn1 : Fcn  Expr=u-1
  Halte Zeit : Subsystem  TreatAsAtomicUnit=on
      settings: RTWFcnNameOpts=Auto  RTWFileNameOpts=Auto
  Logical Operator : Logic  Operator=NOT  Inputs=1
  Mux : Mux  Inputs=2
      settings: DisplayOption=none
  Read : DataStoreRead  DataStoreName=time1  SampleTime=-1
  Relational Operator : RelationalOperator  Operator=>
  "reale Ableitung  " : TransferFcn  Numerator=[1 0]  Denominator=[0.1 1]  AbsoluteTolerance=auto  Realization=auto
  tw2 : ToWorkspace  VariableName=e1  SampleTime=0  SaveFormat=Array
      settings: MaxDataPoints=speicher
  tw3 : ToWorkspace  VariableName=t1  SampleTime=0  SaveFormat=Array
      settings: MaxDataPoints=speicher
  tw4 : ToWorkspace  VariableName=e2  SampleTime=0  SaveFormat=Array
      settings: MaxDataPoints=speicher
  up_l : Outport  Port=1  InitialOutput=0
  wires:
  Logical Operator/1 -> tw2/1, Halte Zeit/Enable
  schaltfreigabe_l/1 -> Logical Operator/1
  Mux/1 -> Fcn/1
  "reale Ableitung  "/1 -> Mux/1
  Fcn1/1 -> Relational Operator/1
  n_Mot/1 -> "reale Ableitung  "/1
  Read/1 -> Relational Operator/2, tw3/1
  Relational Operator/1 -> Mux/2, tw4/1
  Clock1/1 -> Halte Zeit/1(Clock), Fcn1/1
  Fcn/1 -> up_l/1

== system fzgbib/Gangberechnung/Hochschaltung ==
  Motormoment [%] : Inport  Port=1  LatchInput=off
  n_Mot : Inport  Port=2  LatchInput=off
  Gang_i : Inport  Port=3  LatchInput=off
  Kennlinie : Fcn  Expr=30*u+2000
  Relational Operator : RelationalOperator  Operator=>
  Switch : Switch  Threshold=0.5
  u+1 : Fcn  Expr=(u<4)*(u+1)+(u>=4)*4
  Gang_up : Outport  Port=1  InitialOutput=0
  wires:
  Motormoment [%]/1 -> Kennlinie/1
  n_Mot/1 -> Relational Operator/1
  Kennlinie/1 -> Relational Operator/2
  Gang_i/1 -> u+1/1, Switch/3
  u+1/1 -> Switch/1
  Switch/1 -> Gang_up/1
  Relational Operator/1 -> Switch/2

== system fzgbib/Gangberechnung/Rueckrechnung Fahrpedalwert ==
  M_Mot_b : Inport  Port=1  LatchInput=off
  n_Mot : Inport  Port=2  LatchInput=off
  Gain : Gain  Gain=100  Multiplication=Element-wise(K.*u)  SaturateOnIntegerOverflow=on
  Saturation : Saturate  UpperLimit=100  LowerLimit=0  LinearizeAsGain=on
  maximales Motormoment : Lookup  InputValues=n_mot_max  OutputValues=M_mot_max
  u1/u2 : Product  Inputs=*/  Multiplication=Element-wise(.*)  SaturateOnIntegerOverflow=on
  Motormoment [%] : Outport  Port=1  InitialOutput=0
  wires:
  n_Mot/1 -> maximales Motormoment/1
  Saturation/1 -> Motormoment [%]/1
  M_Mot_b/1 -> u1/u2/1
  maximales Motormoment/1 -> u1/u2/2
  u1/u2/1 -> Gain/1
  Gain/1 -> Saturation/1

== system fzgbib/Gangberechnung/Rueckschaltung ==
  Motormoment [%] : Inport  Port=1  LatchInput=off
  n_Mot : Inport  Port=2  LatchInput=off
  Gang_i : Inport  Port=3  LatchInput=off
  Fcn1 : Fcn  Expr=(u>1)*(u-1)+(u<=1)*1
  Kennlinie : Fcn  Expr=28*u+1200
  Relational Operator : RelationalOperator  Operator=<
  Switch : Switch  Threshold=0.5
  Gang_down : Outport  Port=1  InitialOutput=0
  wires:
  Motormoment [%]/1 -> Kennlinie/1
  Kennlinie/1 -> Relational Operator/2
  n_Mot/1 -> Relational Operator/1
  Relational Operator/1 -> Switch/2
  Fcn1/1 -> Switch/1
  Gang_i/1 -> Switch/3, Fcn1/1
  Switch/1 -> Gang_down/1

== system fzgbib/GeschwindigkeitsRegelung/Regler ==
  d_v : Inport  Port=1  LatchInput=off
  Integrator : Integrator  ExternalReset=none  InitialConditionSource=internal  InitialCondition=0  LimitOutput=on  UpperSaturationLimit=2000  LowerSaturationLimit=-2000  ShowSaturationPort=off  ShowStatePort=off  AbsoluteTolerance=auto
  P_Anteil : Gain  Gain=p_anteil  Multiplication=Element-wise(K.*u)  SaturateOnIntegerOverflow=on
  Sum : Sum  Inputs=++  SaturateOnIntegerOverflow=on
  Terminator : Terminator
  "m/s -> km/h1" : Gain  Gain=100  Multiplication=Element-wise(K.*u)  SaturateOnIntegerOverflow=on
  "u_R " : Outport  Port=1  InitialOutput=0
  wires:
  d_v/1 -> "m/s -> km/h1"/1, P_Anteil/1
  "m/s -> km/h1"/1 -> Integrator/1
  P_Anteil/1 -> Sum/1
  Sum/1 -> "u_R "/1
  Integrator/1 -> Terminator/1

== system fzgbib/GeschwindigkeitsRegelung/Stoergroessenkompensation ==
  v_Fzg : Inport  Port=1  LatchInput=off
  v_soll : Inport  Port=2  LatchInput=off
  GR_aktiv_l : Inport  Port=3  LatchInput=off
  Luft- und Rollwiderstand : Subsystem
      settings: RTWFcnNameOpts=Auto  RTWFileNameOpts=Auto
  P-Anteil : Gain  Gain=3000  Multiplication=Element-wise(K.*u)  SaturateOnIntegerOverflow=on
  P-Anteil1 : Gain  Gain=m_Fzg  Multiplication=Element-wise(K.*u)  SaturateOnIntegerOverflow=on
  Sollverhalten Fahrzeug mit P-Regler1 : Subsystem
      settings: RTWFcnNameOpts=Auto  RTWFileNameOpts=Auto
  Sum : Sum  Inputs=2  SaturateOnIntegerOverflow=on
  Sum1 : Sum  Inputs=2  SaturateOnIntegerOverflow=on
  Sum2 : Sum  Inputs=+-  SaturateOnIntegerOverflow=on
  r_dyn : Gain  Gain=r_dyn  Multiplication=Element-wise(K.*u)  SaturateOnIntegerOverflow=on
  reale Ableitung : TransferFcn  Numerator=[1 0]  Denominator=[0.5 1]  AbsoluteTolerance=auto  Realization=auto
  tw5 : ToWorkspace  VariableName=v_Fzg_S  SampleTime=0  SaveFormat=Array
      settings: MaxDataPoints=speicher
  tw8 : ToWorkspace  VariableName=S2  SampleTime=0  SaveFormat=Array
      settings: MaxDataPoints=speicher
  tw9 : ToWorkspace  VariableName=S1  SampleTime=0  SaveFormat=Array
      settings: MaxDataPoints=speicher
  u_s : Outport  Port=1  InitialOutput=0
  wires:
  Sum/1 -> u_s/1
  v_Fzg/1 -> Luft- und Rollwiderstand/1(v_Fzg), Sum2/2, Sollverhalten Fahrzeug mit P-Regler1/2(v_Fzg)
  Sum2/1 -> P-Anteil/1, reale Ableitung/1
  v_soll/1 -> Sollverhalten Fahrzeug mit P-Regler1/1(v_soll)
  reale Ableitung/1 -> r_dyn/1
  GR_aktiv_l/1 -> Sollverhalten Fahrzeug mit P-Regler1/3(GR_aktiv_l)
  r_dyn/1 -> P-Anteil1/1
  Sollverhalten Fahrzeug mit P-Regler1/1(v_Fzg1) -> Sum2/1, tw5/1
  P-Anteil1/1 -> Sum1/1, tw8/1
  P-Anteil/1 -> Sum1/2, tw9/1
  Luft- und Rollwiderstand/1(M_G) -> Sum/1
  Sum1/1 -> Sum/2

== system fzgbib/StellgroessenBerechnung BeschleunigungsBegrenzung/Oneway-Filter ==
  note: 21.5.1997/Hoetzer/FKFS
  in : Inport  Port=1  LatchInput=off
  1/T : Fcn  Expr=1/u
  Fcn : Fcn  Expr=u[1]<-0.01
  Fcn1 : Fcn  Expr=u[1]<0.01
  Grenze3 : Constant  Value=zk
  Grenze4 : Constant  Value=0.1
  Integrator : Integrator  ExternalReset=none  InitialConditionSource=internal  InitialCondition=0  LimitOutput=off  UpperSaturationLimit=inf  LowerSaturationLimit=-inf  ShowSaturationPort=off  ShowStatePort=off  AbsoluteTolerance=auto
  Logical Operator : Logic  Operator=OR  Inputs=2
  Logical Operator1 : Logic  Operator=AND  Inputs=2
  Product : Product  Inputs=2  Multiplication=Element-wise(.*)  SaturateOnIntegerOverflow=on
  Reglerabweichung : Sum  Inputs=-+  SaturateOnIntegerOverflow=on
  Relational Operator1 : RelationalOperator  Operator=>=
  Switch : Switch  Threshold=0.5
  reale Ableitung : TransferFcn  Numerator=[1 0]  Denominator=[0.1 1]  AbsoluteTolerance=auto  Realization=auto
  "out " : Outport  Port=1  InitialOutput=0
  wires:
  Logical Operator1/1 -> Logical Operator/1
  Fcn1/1 -> Logical Operator/2
  Integrator/1 -> "out "/1, Reglerabweichung/1, Relational Operator1/1
  Product/1 -> Integrator/1
  Logical Operator/1 -> Switch/2
  Switch/1 -> 1/T/1
  Reglerabweichung/1 -> Product/1
  1/T/1 -> Product/2
  in/1 -> Reglerabweichung/2, reale Ableitung/1, Fcn1/1, Relational Operator1/2
  Grenze4/1 -> Switch/1
  Grenze3/1 -> Switch/3
  reale Ableitung/1 -> Fcn/1
  Fcn/1 -> Logical Operator1/1
  Relational Operator1/1 -> Logical Operator1/2

== system fzgbib/StellgroessenBerechnung BeschleunigungsBegrenzung/neg. Beschleunigungsbegrenzung ==
  note: Das Bremsmoment wird solange durchgereicht, solange die Beschleunigung > -2 ist.
      | Im anderen Fall wird das in diesem Fall gespeicherte Bremsmoment durchgereicht.
  M_Br_v : Inport  Port=1  LatchInput=off
  a_Fzg_mss : Inport  Port=2  LatchInput=off
  M_Br_n : Inport  Port=3  LatchInput=off
  Constant1 : Constant  Value=a_Fzg_min
  Data Store Memory : DataStoreMemory  DataStoreName=M_Br2  InitialValue=0
  Data Store Read : DataStoreRead  DataStoreName=M_Br2  SampleTime=-1
  Gangspeicher : Memory  X0=1  InheritSampleTime=off
      settings: RTWStateStorageClass=Auto
  Logical Operator : Logic  Operator=OR  Inputs=2
  Logical Operator1 : Logic  Orientation=down  Operator=NOT  Inputs=1
  Relational Operator : RelationalOperator  Operator=>
  Relational Operator1 : RelationalOperator  Operator=<=
  Reset M_Br2 : Subsystem  TreatAsAtomicUnit=on
      settings: RTWFcnNameOpts=Auto  RTWFileNameOpts=Auto
  Switch : Switch  Threshold=0.5
  tw5 : ToWorkspace  VariableName=b_l  SampleTime=0  SaveFormat=Array
      settings: MaxDataPoints=speicher
  tw6 : ToWorkspace  VariableName=M_Br2  SampleTime=0  SaveFormat=Array
      settings: MaxDataPoints=speicher
  tw7 : ToWorkspace  VariableName=M_Br1  SampleTime=0  SaveFormat=Array
      settings: MaxDataPoints=speicher
  M_Br3 : Outport  Port=1  InitialOutput=0
  wires:
  a_Fzg_mss/1 -> Reset M_Br2/2(a_Fzg_mss), Relational Operator/1
  Logical Operator1/1 -> Reset M_Br2/Enable
  Relational Operator/1 -> Logical Operator1/1, Logical Operator/1
  M_Br_v/1 -> Relational Operator1/1, tw7/1, Switch/1
  M_Br_n/1 -> Reset M_Br2/1(M_Br_n)
  Gangspeicher/1 -> tw5/1, Switch/2
  Logical Operator/1 -> Gangspeicher/1
  Data Store Read/1 -> Relational Operator1/2, tw6/1, Switch/3
  Relational Operator1/1 -> Logical Operator/2
  Constant1/1 -> Relational Operator/2
  Switch/1 -> M_Br3/1
